simulink model "CruiseControl"  (Simulink 10.1)
settings: Solver=VariableStepAuto  StartTime=0.0  StopTime=200  RelTol=1e-3
values from neighbouring files (symbols this model uses):
  A = 2.4    [constants2.m]
  a3 = 16    [constants2.m]
  beta = 0.4    [constants2.m]
  cd = 0.32    [constants2.m]
  cr = 0.01    [constants2.m]
  g = 9.8    [constants2.m]
  m = 800    [constants2.m]
  rho = 1.3    [constants2.m]
  tm = 190    [constants2.m]
  wm = 420    [constants2.m]
settings Model: Creator=M. Tilocca  LastModifiedBy=M. Tilocca
settings DataIOCC: SaveFormat=Dataset  ReturnWorkspaceOutputs=on
settings OptimizationCC: LifeSpan=auto
settings DebuggingCC: UnderspecifiedInitializationDetection=Simplified  MergeDetectMultiDrivingBlocksExec=error  SFUnexpectedBacktrackingDiag=error  SFNoUnconditionalDefaultTransitionDiag=error  SFExecutionAtInitializationDiag=warning  ArithmeticOperatorsInVariantConditions=error
settings HardwareCC: ProdBitPerPointer=64  ProdBitPerSizeT=64  ProdBitPerPtrDiffT=64  ProdLargestAtomicFloat=Float  ProdIntDivRoundTo=Zero  ProdEndianess=LittleEndian  ProdWordSize=64  ProdHWDeviceType=Intel->x86-64 (Windows64)
settings ModelReferenceCC: PropagateSignalLabelsOutOfModel=on
settings SFSimCC: SimUseLocalCustomCode=on  CustomCodeUndefinedFunction=FilterOut
settings RTWCC: RTWUseLocalCustomCode=on
settings CodeAppCC: StateflowObjectComments=off
settings GRTTargetCC: TargetLangStandard=C99 (ISO)  CombineOutputUpdateFcns=on  GRTInterface=off
settings ConfigComp: CovMetricSettings=dwe  CovHtmlReporting=off  CovSaveCumulativeToWorkspaceVar=off  CovSaveSingleToWorkspaceVar=off  CovExternalEMLEnable=on

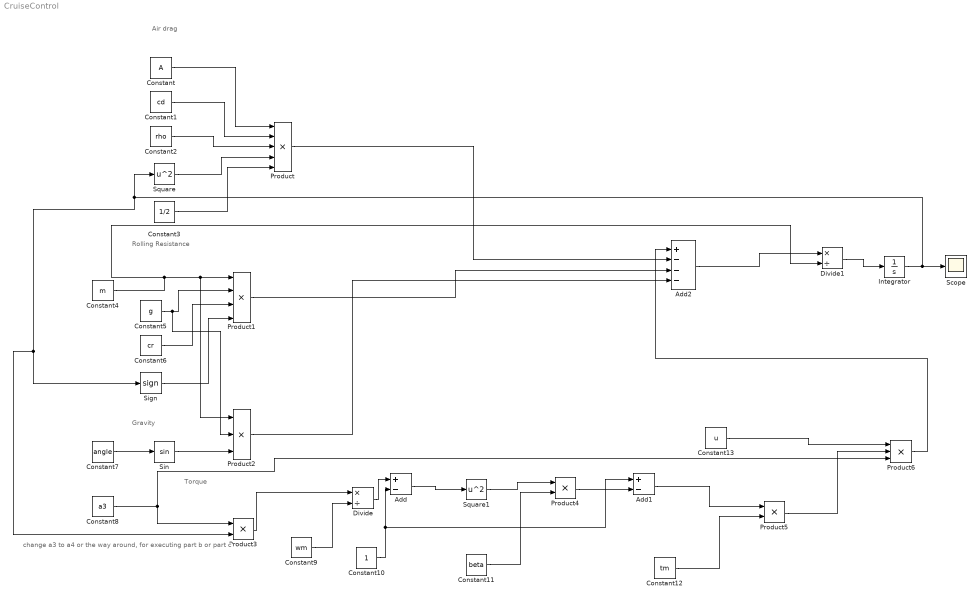
== system CruiseControl ==
  note: change a3 to a4 or the way around, for executing part b or part c
  note: Torque
  note: Rolling Resistance
  note: Air drag
  note: Gravity
  Add : Sum  Inputs=+-
  Add1 : Sum  Inputs=+-
  Add2 : Sum  Inputs=+---
  Constant : Constant  Value=A
  Constant1 : Constant  Value=cd
  Constant10 : Constant
  Constant11 : Constant  Value=beta
  Constant12 : Constant  Value=tm
  Constant13 : Constant  Value=u
  Constant2 : Constant  Value=rho
  Constant3 : Constant  Value=1/2
  Constant4 : Constant  Value=m
  Constant5 : Constant  Value=g
  Constant6 : Constant  Value=cr
  Constant7 : Constant  Value=angle
  Constant8 : Constant  Value=a3
  Constant9 : Constant  Value=wm
  Divide : Product  Inputs=*/
  Divide1 : Product  Inputs=*/
  Integrator : Integrator
  Product : Product  Inputs=5
  Product1 : Product  Inputs=4
  Product2 : Product  Inputs=3
  Product3 : Product
  Product4 : Product
  Product5 : Product
  Product6 : Product  Inputs=3
  Scope : Scope
  Sign : Signum
  Sin : Trigonometry
  Square : Math  Operator=square  SaturateOnIntegerOverflow=on
  Square1 : Math  Operator=square  SaturateOnIntegerOverflow=on
  wires:
  Constant9/1 -> Divide/2
  Constant11/1 -> Product4/2
  Product3/1 -> Divide/1
  Sign/1 -> Product1/4
  Constant5/1 -> Product2/2, Product1/2
  Constant8/1 -> Product3/1, Product6/3
  Constant2/1 -> Product/3
  Constant/1 -> Product/1
  Constant10/1 -> Add1/1, Add/2
  Constant4/1 -> Product1/1, Product2/1, Divide1/2
  Constant1/1 -> Product/2
  Square1/1 -> Product4/1
  Constant3/1 -> Product/5
  Add/1 -> Square1/1
  Constant6/1 -> Product1/3
  Sin/1 -> Product2/3
  Constant7/1 -> Sin/1
  Divide/1 -> Add/1
  Square/1 -> Product/4
  Add1/1 -> Product5/1
  Constant12/1 -> Product5/2
  Product5/1 -> Product6/2
  Constant13/1 -> Product6/1
  Add2/1 -> Divide1/1
  Divide1/1 -> Integrator/1
  Integrator/1 -> Square/1, Product3/2, Sign/1, Scope/1
  Product6/1 -> Add2/1
  Product/1 -> Add2/2
  Product1/1 -> Add2/3
  Product2/1 -> Add2/4
  Product4/1 -> Add1/2
